simulink library "lib_power_bus"  (Simulink 4.00)
undefined symbols (not defined in the file or in its folder): acc_elec_eff, acc_elec_pwr, cs_hi_soc, cs_lo_soc, ess_on
libraries: sub_lib_models x2
settings Model: LastModifiedBy=mokeefe
settings Model: ModifiedComment=|
  | mokeefe -- Thu Apr 18 08:38:09 2002 -- Version 1.10
  | saving the model:
  | o "without the model browser open"
  | o with only top-level screen visible
  | o with "fit to view" enabled
  | o with "status bar" off and "toolbar" off
  | o with "prompt to update model history with each save" on
settings Model: ModifiedHistory=|
  | mokeefe -- Thu Apr 18 08:38:09 2002 -- Version 1.10
  | saving the model:
  | o "without the model browser open"
  | o with only top-level screen visible
  | o with "fit to view" enabled
  | o with "status bar" off and "toolbar" off
  | o with "prompt to update model history with each save" on

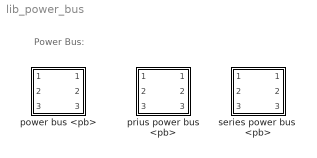
== system lib_power_bus ==
  note: Power Bus:
  power bus <pb> : Subsystem
      settings: RTWFcnNameOpts=Auto  RTWFileNameOpts=Auto
      mask Display: image(imread('bdi_pb.jpg'))
  prius power bus <pb> : Subsystem
      settings: RTWFcnNameOpts=Auto  RTWFileNameOpts=Auto
      mask Display: image(imread('bdi_pb.jpg'))
  series power bus  <pb> : Subsystem
      settings: RTWFcnNameOpts=Auto  RTWFileNameOpts=Auto
      mask Display: image(imread('bdi_pb.jpg'))

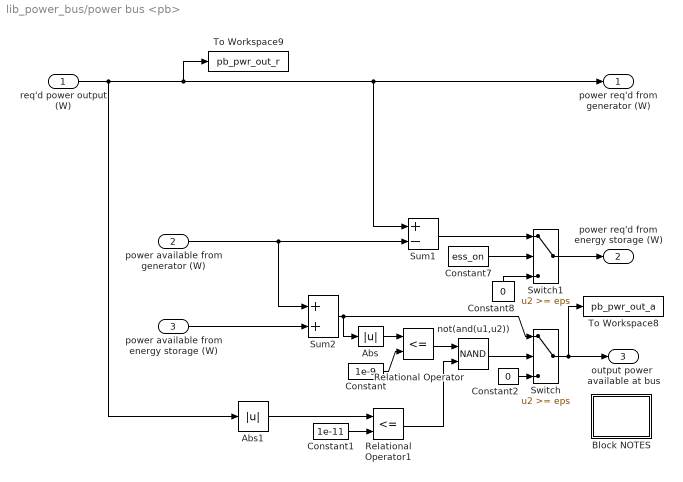
== system lib_power_bus/power bus <pb> ==
  req'd power output (W) : Inport  Port=1  LatchInput=off
  power available from generator (W) : Inport  Port=2  LatchInput=off
  power available from energy storage (W) : Inport  Port=3  LatchInput=off
  Abs : Abs  SaturateOnIntegerOverflow=on
  Abs1 : Abs  SaturateOnIntegerOverflow=on
  Block NOTES : Subsystem
      settings: RTWFcnNameOpts=Auto  RTWFileNameOpts=Auto
      mask Display: disp('Block\nNOTES')
  Constant : Constant  Value=1e-9
  Constant1 : Constant  Value=1e-11
  Constant2 : Constant  Value=0
  Constant7 : Constant  Value=ess_on
  Constant8 : Constant  Orientation=up  Value=0
  Relational Operator : RelationalOperator  Operator=<=
  Relational Operator1 : RelationalOperator  Operator=<=
  Sum1 : Sum  Inputs=+-  SaturateOnIntegerOverflow=on
  Sum2 : Sum  Inputs=++  SaturateOnIntegerOverflow=on
  Switch : Switch  Threshold=eps
  Switch1 : Switch  Threshold=eps
  To Workspace8 : ToWorkspace  VariableName=pb_pwr_out_a  SampleTime=-1  SaveFormat=Array
  To Workspace9 : ToWorkspace  VariableName=pb_pwr_out_r  SampleTime=-1  SaveFormat=Array
  not(and(u1,u2)) : Logic  Operator=NAND  Inputs=2
  power req'd from generator (W) : Outport  Port=1
  power req'd from energy storage (W) : Outport  Port=2
  output power  available at bus : Outport  Port=3
  wires:
  req'd power output (W)/1 -> Abs1/1, To Workspace9/1, Sum1/1, power req'd from generator (W)/1
  power available from generator (W)/1 -> Sum2/1, Sum1/2
  Relational Operator/1 -> not(and(u1,u2))/1
  Constant2/1 -> Switch/3
  not(and(u1,u2))/1 -> Switch/2
  Relational Operator1/1 -> not(and(u1,u2))/2
  Abs1/1 -> Relational Operator1/1
  Constant1/1 -> Relational Operator1/2
  Switch/1 -> To Workspace8/1, output power  available at bus/1
  Sum2/1 -> Abs/1, Switch/1
  Abs/1 -> Relational Operator/1
  Constant/1 -> Relational Operator/2
  Sum1/1 -> Switch1/1
  Switch1/1 -> power req'd from energy storage (W)/1
  Constant7/1 -> Switch1/2
  Constant8/1 -> Switch1/3
  power available from energy storage (W)/1 -> Sum2/2

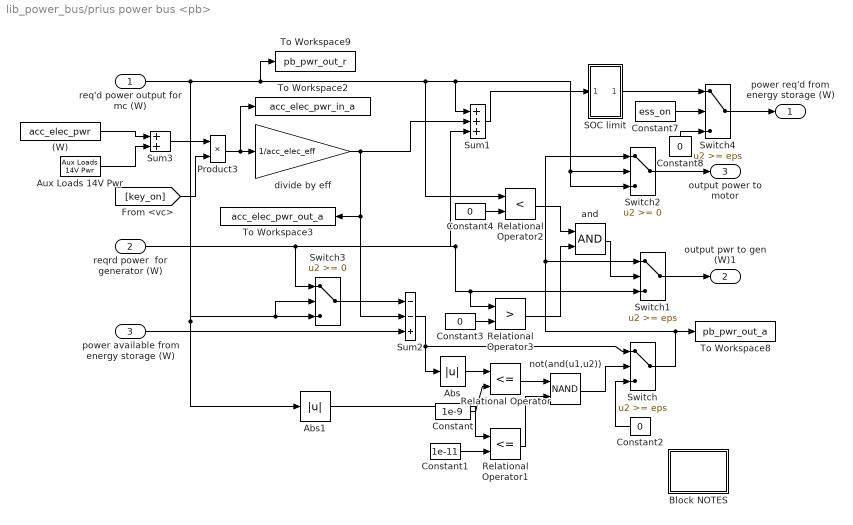
== system lib_power_bus/prius power bus <pb> ==
  req'd power output for mc (W) : Inport  Port=1  LatchInput=off
  reqrd power  for generator (W) : Inport  Port=2  LatchInput=off
  power available from energy storage (W) : Inport  Port=3  LatchInput=off
  (W) : Constant  Value=acc_elec_pwr
  Abs : Abs  SaturateOnIntegerOverflow=on
  Abs1 : Abs  SaturateOnIntegerOverflow=on
  Aux Loads 14V Pwr : sub_lib_models/Aux Loads 14V Pwr
      settings: RTWFcnNameOpts=Auto  RTWFileNameOpts=Auto
  Block NOTES : Subsystem
      settings: RTWFcnNameOpts=Auto  RTWFileNameOpts=Auto
      mask Display: disp('Block\nNOTES')
  Constant : Constant  Value=1e-9
  Constant1 : Constant  Value=1e-11
  Constant2 : Constant  Orientation=left  Value=0
  Constant3 : Constant  Value=0
  Constant4 : Constant  Value=0
  Constant7 : Constant  Value=ess_on
  Constant8 : Constant  Orientation=up  Value=0
  Product3 : Product  Inputs=2  Multiplication=Element-wise(.*)  SaturateOnIntegerOverflow=on
  Relational Operator : RelationalOperator  Operator=<=
  Relational Operator1 : RelationalOperator  Operator=<=
  Relational Operator2 : RelationalOperator  Operator=<
  Relational Operator3 : RelationalOperator  Operator=>
  SOC limit : Subsystem
      settings: RTWFcnNameOpts=Auto  RTWFileNameOpts=Auto
  Sum1 : Sum  Inputs=+++  SaturateOnIntegerOverflow=on
  Sum2 : Sum  Inputs=--+  SaturateOnIntegerOverflow=on
  Sum3 : Sum  Inputs=++  SaturateOnIntegerOverflow=on
  Switch : Switch  Threshold=eps
  Switch1 : Switch  Threshold=eps
  Switch2 : Switch  Threshold=0
  Switch3 : Switch  Threshold=0
  Switch4 : Switch  Threshold=eps
  To Workspace2 : ToWorkspace  VariableName=acc_elec_pwr_in_a  SampleTime=-1  SaveFormat=Array
  To Workspace3 : ToWorkspace  VariableName=acc_elec_pwr_out_a  SampleTime=-1  SaveFormat=Array
  To Workspace8 : ToWorkspace  VariableName=pb_pwr_out_a  SampleTime=-1  SaveFormat=Array
  To Workspace9 : ToWorkspace  VariableName=pb_pwr_out_r  SampleTime=-1  SaveFormat=Array
  and : Logic  Operator=AND  Inputs=2
  divide by eff : Gain  Gain=1/acc_elec_eff  Multiplication=Element-wise(K.*u)  SaturateOnIntegerOverflow=on
  not(and(u1,u2)) : Logic  Operator=NAND  Inputs=2
  power req'd from energy storage (W) : Outport  Port=1
  output pwr to gen (W)1 : Outport  Port=2
  output power to motor : Outport  Port=3
  wires:
  and/1 -> Switch1/2
  Relational Operator3/1 -> and/2
  Relational Operator2/1 -> and/1
  Constant4/1 -> Relational Operator2/2
  Constant3/1 -> Relational Operator3/2
  Constant8/1 -> Switch4/3
  Constant7/1 -> Switch4/2
  Switch4/1 -> power req'd from energy storage (W)/1
  SOC limit/1(limited pwr req from ess (W)) -> Switch4/1
  Sum1/1 -> SOC limit/1(pwr req to  ess)
  Switch/1 -> Switch2/1, Switch1/1, To Workspace8/1
  reqrd power  for generator (W)/1 -> Switch3/1, Switch1/3, Relational Operator3/1, Sum1/3
  Switch3/1 -> Sum2/1
  Switch1/1 -> output pwr to gen (W)1/1
  Switch2/1 -> output power to motor/1
  Constant1/1 -> Relational Operator1/2
  Relational Operator1/1 -> not(and(u1,u2))/2
  Abs1/1 -> Relational Operator1/1
  Constant/1 -> Relational Operator/2
  Relational Operator/1 -> not(and(u1,u2))/1
  not(and(u1,u2))/1 -> Switch/2
  Constant2/1 -> Switch/3
  Abs/1 -> Relational Operator/1
  Sum2/1 -> Switch/1, Abs/1
  power available from energy storage (W)/1 -> Sum2/3
  Product3/1 -> To Workspace2/1, divide by eff/1
  divide by eff/1 -> Sum1/2, To Workspace3/1, Sum2/2
  [key_on] -> Product3/2
  req'd power output for mc (W)/1 -> Switch3/2, Switch3/3, Abs1/1, Relational Operator2/1, Switch2/2, Switch2/3, Sum1/1, To Workspace9/1
  Sum3/1 -> Product3/1
  (W)/1 -> Sum3/1
  Aux Loads 14V Pwr/1 -> Sum3/2

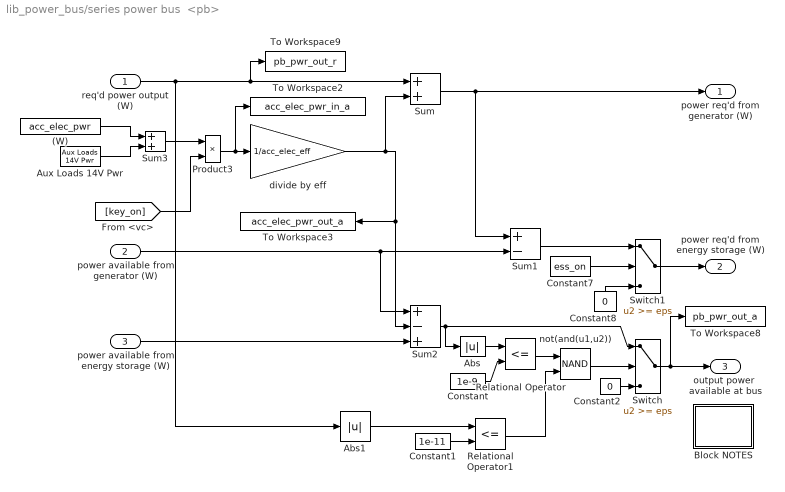
== system lib_power_bus/series power bus  <pb> ==
  req'd power output (W) : Inport  Port=1  LatchInput=off
  power available from generator (W) : Inport  Port=2  LatchInput=off
  power available from energy storage (W) : Inport  Port=3  LatchInput=off
  (W) : Constant  Value=acc_elec_pwr
  Abs : Abs  SaturateOnIntegerOverflow=on
  Abs1 : Abs  SaturateOnIntegerOverflow=on
  Aux Loads 14V Pwr : sub_lib_models/Aux Loads 14V Pwr
      settings: RTWFcnNameOpts=Auto  RTWFileNameOpts=Auto
  Block NOTES : Subsystem
      settings: RTWFcnNameOpts=Auto  RTWFileNameOpts=Auto
      mask Display: disp('Block\nNOTES')
  Constant : Constant  Value=1e-9
  Constant1 : Constant  Value=1e-11
  Constant2 : Constant  Value=0
  Constant7 : Constant  Value=ess_on
  Constant8 : Constant  Orientation=up  Value=0
  Product3 : Product  Inputs=2  Multiplication=Element-wise(.*)  SaturateOnIntegerOverflow=on
  Relational Operator : RelationalOperator  Operator=<=
  Relational Operator1 : RelationalOperator  Operator=<=
  Sum : Sum  Inputs=++  SaturateOnIntegerOverflow=on
  Sum1 : Sum  Inputs=+-  SaturateOnIntegerOverflow=on
  Sum2 : Sum  Inputs=+-+  SaturateOnIntegerOverflow=on
  Sum3 : Sum  Inputs=++  SaturateOnIntegerOverflow=on
  Switch : Switch  Threshold=eps
  Switch1 : Switch  Threshold=eps
  To Workspace2 : ToWorkspace  VariableName=acc_elec_pwr_in_a  SampleTime=-1  SaveFormat=Array
  To Workspace3 : ToWorkspace  VariableName=acc_elec_pwr_out_a  SampleTime=-1  SaveFormat=Array
  To Workspace8 : ToWorkspace  VariableName=pb_pwr_out_a  SampleTime=-1  SaveFormat=Array
  To Workspace9 : ToWorkspace  VariableName=pb_pwr_out_r  SampleTime=-1  SaveFormat=Array
  divide by eff : Gain  Gain=1/acc_elec_eff  Multiplication=Element-wise(K.*u)  SaturateOnIntegerOverflow=on
  not(and(u1,u2)) : Logic  Operator=NAND  Inputs=2
  power req'd from generator (W) : Outport  Port=1
  power req'd from energy storage (W) : Outport  Port=2
  output power  available at bus : Outport  Port=3
  wires:
  Constant8/1 -> Switch1/3
  Constant7/1 -> Switch1/2
  Switch1/1 -> power req'd from energy storage (W)/1
  Sum1/1 -> Switch1/1
  Constant/1 -> Relational Operator/2
  Abs/1 -> Relational Operator/1
  Sum2/1 -> Switch/1, Abs/1
  Switch/1 -> output power  available at bus/1, To Workspace8/1
  Constant1/1 -> Relational Operator1/2
  Abs1/1 -> Relational Operator1/1
  Relational Operator1/1 -> not(and(u1,u2))/2
  not(and(u1,u2))/1 -> Switch/2
  Constant2/1 -> Switch/3
  power available from energy storage (W)/1 -> Sum2/3
  Relational Operator/1 -> not(and(u1,u2))/1
  power available from generator (W)/1 -> Sum1/2, Sum2/1
  Product3/1 -> To Workspace2/1, divide by eff/1
  [key_on] -> Product3/2
  Sum/1 -> power req'd from generator (W)/1, Sum1/1
  req'd power output (W)/1 -> To Workspace9/1, Sum/1, Abs1/1
  divide by eff/1 -> Sum/2, Sum2/2, To Workspace3/1
  Sum3/1 -> Product3/1
  (W)/1 -> Sum3/1
  Aux Loads 14V Pwr/1 -> Sum3/2

== system lib_power_bus/power bus <pb>/Block NOTES ==
  note: This power bus requires power from (or distributes power to)
      | the generator first, taking the balance from the energy
      | storage system.

== system lib_power_bus/prius power bus <pb>/Block NOTES ==
  note: This power bus requires power from (or distributes power to)
      | the generator first, taking the balance from the energy
      | storage system.

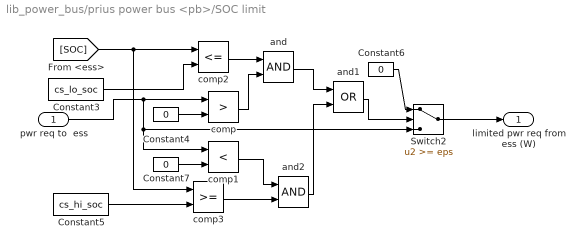
== system lib_power_bus/prius power bus <pb>/SOC limit ==
  pwr req to  ess : Inport  Port=1  LatchInput=off
  Constant3 : Constant  Value=cs_lo_soc
  Constant4 : Constant  Value=0
  Constant5 : Constant  Value=cs_hi_soc
  Constant6 : Constant  Value=0
  Constant7 : Constant  Value=0
  Switch2 : Switch  Threshold=eps
  and : Logic  Operator=AND  Inputs=2
  and1 : Logic  Operator=OR  Inputs=2
  and2 : Logic  Operator=AND  Inputs=2
  comp : RelationalOperator  Operator=>
  comp1 : RelationalOperator  Operator=<
  comp2 : RelationalOperator  Operator=<=
  comp3 : RelationalOperator  Operator=>=
  limited pwr req from ess (W) : Outport  Port=1  InitialOutput=0
  wires:
  Switch2/1 -> limited pwr req from ess (W)/1
  comp2/1 -> and/1
  Constant3/1 -> comp2/2
  and/1 -> and1/1
  and1/1 -> Switch2/2
  [SOC] -> comp2/1, comp3/1
  comp/1 -> and/2
  comp1/1 -> and2/1
  pwr req to  ess/1 -> comp/1, comp1/1, Switch2/3
  Constant6/1 -> Switch2/1
  Constant5/1 -> comp3/2
  comp3/1 -> and2/2
  and2/1 -> and1/2
  Constant4/1 -> comp/2
  Constant7/1 -> comp1/2

== system lib_power_bus/series power bus  <pb>/Block NOTES ==
  note: This power bus requires power from (or distributes power to)
      | the generator first, taking the balance from the energy
      | storage system.
